simulink model "Continuous_UIO"  (R2021a)
settings: Solver=VariableStepAuto  StartTime=0.0  StopTime=10.0  RelTol=1e-3
values from neighbouring files (symbols this model uses):
  B2 = [4 ... (first row only)    [FunWork5.m]
  D2 = [0 0 ... (first row only)    [FunWork5.m]
  K = Z*S^-1    [FunWork5.m]
  L = X'    [FunWork5.m]
  M = B2*pinv(C*B2)    [FunWork5.m]
  q0 = pi*([x0.x;x0.theta1;x0.theta2;x0.x_dot;x0.theta1_dot;x0.theta2_dot]-x_e)    [FunWork5.m]
undefined symbols (not defined in the file or in its folder): A, B, C, u_e, x0, x_e
libraries: vrlib x2, aerolibanimutils x1, dspvision x1
settings Model: Creator=vicen  LastModifiedBy=vicen

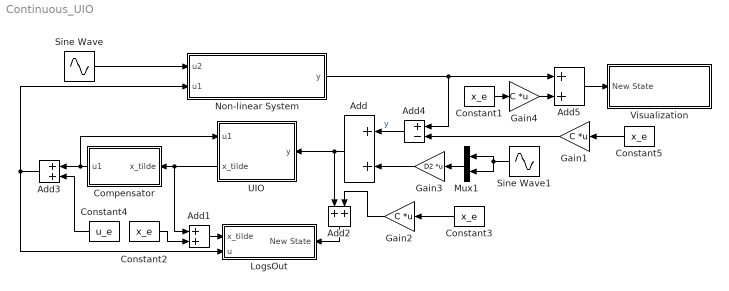
== system Continuous_UIO ==
  Add{,1..3,5} (5 alike) : Sum
  Add4 : Sum  Inputs=+-
  Compensator : Subsystem
  Constant{1..3,5} (4 alike) : Constant  Value=x_e
  Constant4 : Constant  Value=u_e
  Gain1 : Gain  Gain=C  Multiplication=Matrix(K*u)
  Gain2 : Gain  Gain=C  Multiplication=Matrix(K*u)
  Gain3 : Gain  Gain=D2  Multiplication=Matrix(K*u)
  Gain4 : Gain  Gain=C  Multiplication=Matrix(K*u)
  LogsOut : Subsystem
      settings: PortSchema="{\"entries\":[{\"content\":{\"sides\":[{\"content\":{\"connectorIds\":[\"In1\",\"In2\"]},\"type\":\"ConnectorPlacement.EquallySpacedRectSide\",\"uuid\":\"a6e5c360-9678-424a-aca2-159feab9ca2f\"},{\"content\":{\"connectorIds\":[\"In3\"],\"side\":\"RIGHT\"},\"type\":\"ConnectorPlacement.EquallySpacedRectSide\",\"uuid\":\"87be8f2e-6499-443d-a388-19aeb21b3c40\"},{\"content\":{\"connectorIds\":[],\"side\":\"TOP\"},\"type\":\"ConnectorPlacement.EquallySpacedRectSide\",\"uuid\":\"16b12663-65e7-4c0d-a383-2b4d1475174c\"}]},\"type\":\"ConnectorPlacement.EquallySpacedConnector\",\"uuid\":\"7c26d127-e336-47cd-9b3d-f4001f849349\"}],\"packageUris\":[\"http://schema.mathworks.com/mf0/Connector/R2020b\"],\"version\":\"1.0\"}"
  Mux1 : Mux  Inputs=2
  Non-linear System : Subsystem
  Sine Wave : Sin  Amplitude=.001  SampleTime=0
  Sine Wave1 : Sin  Amplitude=.001  SampleTime=0
  UIO : Subsystem
      settings: PortSchema="{\"entries\":[{\"content\":{\"sides\":[{\"content\":{\"connectorIds\":[\"In1\"]},\"type\":\"ConnectorPlacement.EquallySpacedRectSide\",\"uuid\":\"e0fdc8c6-333c-4d3c-a4a6-b3300e16a61f\"},{\"content\":{\"connectorIds\":[\"In2\",\"Out1\"],\"side\":\"RIGHT\"},\"type\":\"ConnectorPlacement.EquallySpacedRectSide\",\"uuid\":\"dbf4194e-4b72-4f2d-9e59-4d14081d6aaf\"},{\"content\":{\"connectorIds\":[],\"side\":\"TOP\"},\"type\":\"ConnectorPlacement.EquallySpacedRectSide\",\"uuid\":\"2ba0a26c-1285-47ee-b6f8-efca2049e722\"}]},\"type\":\"ConnectorPlacement.EquallySpacedConnector\",\"uuid\":\"ed710a6f-1694-499a-b832-87fa0fefc432\"}],\"packageUris\":[\"http://schema.mathworks.com/mf0/Connector/R2020b\"],\"version\":\"1.0\"}"
  Visualization : Subsystem
  wires:
  UIO/1(x_tilde) -> Compensator/1(x_tilde), Add1/1
  Gain3/1 -> Add/2
  Sine Wave1/1 -> Mux1/2, Mux1/1
  Sine Wave/1 -> Non-linear System/1(u2)
  Non-linear System/1(y) -> Add4/1, Add5/1
  Constant2/1 -> Add1/2
  Add1/1 -> LogsOut/1(x_tilde)
  Add/1 -> UIO/1(y), Add2/1
  Constant3/1 -> Gain2/1
  Add2/1 -> LogsOut/3(New State)
  Constant4/1 -> Add3/2
  Compensator/1(u1) -> Add3/1, UIO/2(u1)
  Add3/1 -> Non-linear System/2(u1), LogsOut/2(u)
  Constant5/1 -> Gain1/1
  Add4/1 -> Add/1  "y"
  Gain1/1 -> Add4/2
  Mux1/1 -> Gain3/1
  Gain2/1 -> Add2/2
  Gain4/1 -> Add5/2
  Constant1/1 -> Gain4/1
  Add5/1 -> Visualization/1(New State)

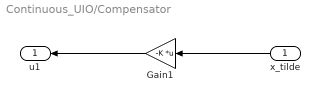
== system Continuous_UIO/Compensator ==
  x_tilde : Inport
  Gain1 : Gain  Gain=-K  Multiplication=Matrix(K*u)
  u1 : Outport
  wires:
  x_tilde/1 -> Gain1/1
  Gain1/1 -> u1/1

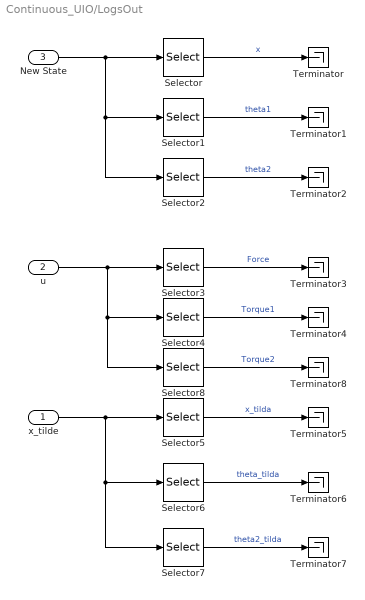
== system Continuous_UIO/LogsOut ==
  x_tilde : Inport
  u : Inport  Port=2
  New State : Inport  Port=3
  Selector : Selector  InputPortWidth=3  IndexOptions=Index vector (dialog)  Indices=1  OutputSizes=1
  Selector1 : Selector  InputPortWidth=3  IndexOptions=Index vector (dialog)  Indices=2  OutputSizes=1
  Selector2 : Selector  InputPortWidth=3  IndexOptions=Index vector (dialog)  Indices=3  OutputSizes=1
  Selector3 : Selector  InputPortWidth=3  IndexOptions=Index vector (dialog)  Indices=1  OutputSizes=1
  Selector4 : Selector  InputPortWidth=3  IndexOptions=Index vector (dialog)  Indices=2  OutputSizes=1
  Selector5 : Selector  InputPortWidth=6  IndexOptions=Index vector (dialog)  Indices=1  OutputSizes=1
  Selector6 : Selector  InputPortWidth=6  IndexOptions=Index vector (dialog)  Indices=2  OutputSizes=1
  Selector7 : Selector  InputPortWidth=6  IndexOptions=Index vector (dialog)  Indices=3  OutputSizes=1
  Selector8 : Selector  InputPortWidth=3  IndexOptions=Index vector (dialog)  Indices=3  OutputSizes=1
  Terminator{,1..8} (9 alike) : Terminator
  wires:
  Selector/1 -> Terminator/1  "x"
  Selector1/1 -> Terminator1/1  "theta1"
  Selector2/1 -> Terminator2/1  "theta2"
  New State/1 -> Selector2/1, Selector1/1, Selector/1
  u/1 -> Selector8/1, Selector4/1, Selector3/1
  Selector4/1 -> Terminator4/1  "Torque1"
  Selector3/1 -> Terminator3/1  "Force"
  x_tilde/1 -> Selector5/1, Selector7/1, Selector6/1
  Selector5/1 -> Terminator5/1  "x_tilda"
  Selector6/1 -> Terminator6/1  "theta_tilda"
  Selector7/1 -> Terminator7/1  "theta2_tilda"
  Selector8/1 -> Terminator8/1  "Torque2"

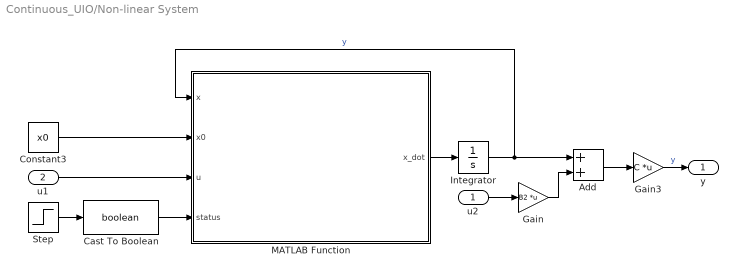
== system Continuous_UIO/Non-linear System ==
  u2 : Inport
  u1 : Inport  Port=2
  Add : Sum
  Cast To Boolean : DataTypeConversion  OutDataTypeStr=boolean
  Constant3 : Constant  Value=x0  VectorParams1D=off  OutDataTypeStr=Bus: State_bus
  Gain : Gain  Gain=B2  Multiplication=Matrix(K*u)
  Gain3 : Gain  Gain=C  Multiplication=Matrix(K*u)
  Integrator : Integrator  InitialCondition=[x0.x;x0.theta1;x0.theta2;x0.x_dot;x0.theta1_dot;x0.theta2_dot]
  MATLAB Function : MATLAB Function  TreatAsAtomicUnit=on
  Step : Step  Time=.001  SampleTime=0
  y : Outport
  wires:
  u1/1 -> MATLAB Function/3(u)
  Step/1 -> Cast To Boolean/1
  Cast To Boolean/1 -> MATLAB Function/4(status)
  Integrator/1 -> Add/1, MATLAB Function/1(x)  "y"
  Constant3/1 -> MATLAB Function/2(x0)
  u2/1 -> Gain/1
  Gain/1 -> Add/2
  MATLAB Function/1(x_dot) -> Integrator/1
  Add/1 -> Gain3/1
  Gain3/1 -> y/1  "y"

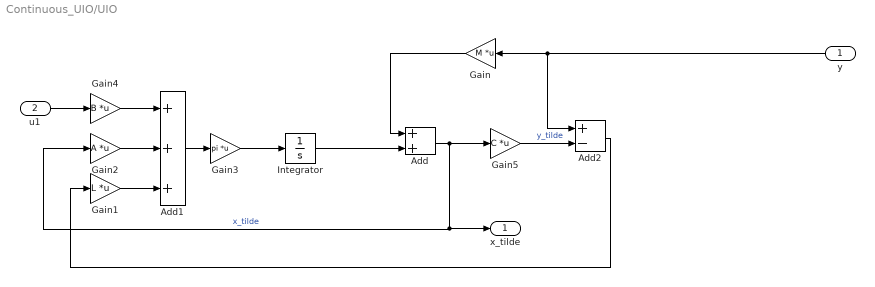
== system Continuous_UIO/UIO ==
  y : Inport
  u1 : Inport  Port=2
  Add : Sum
  Add1 : Sum  Inputs=+++
  Add2 : Sum  Inputs=+-
  Gain : Gain  Gain=M  Multiplication=Matrix(K*u)
  Gain1 : Gain  Gain=L  Multiplication=Matrix(K*u)
  Gain2 : Gain  Gain=A  Multiplication=Matrix(K*u)
  Gain3 : Gain  Gain=pi  Multiplication=Matrix(K*u)
  Gain4 : Gain  Gain=B  Multiplication=Matrix(K*u)
  Gain5 : Gain  Gain=C  Multiplication=Matrix(K*u)
  Integrator : Integrator  InitialCondition=q0
  x_tilde : Outport
  wires:
  Gain/1 -> Add/1
  y/1 -> Gain/1, Add2/1
  u1/1 -> Gain4/1
  Gain4/1 -> Add1/1
  Add1/1 -> Gain3/1
  Integrator/1 -> Add/2
  Add/1 -> Gain2/1, x_tilde/1, Gain5/1  "x_tilde"
  Gain5/1 -> Add2/2  "y_tilde"
  Add2/1 -> Gain1/1
  Gain2/1 -> Add1/2
  Gain1/1 -> Add1/3
  Gain3/1 -> Integrator/1

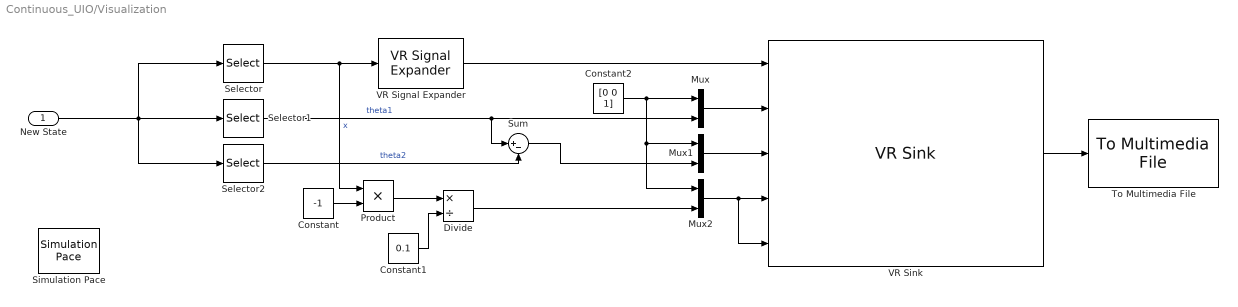
== system Continuous_UIO/Visualization ==
  New State : Inport
  Constant : Constant  Value=-1
  Constant1 : Constant  Value=0.1
  Constant2 : Constant  Value=[0 0 1]
  Divide : Product  Inputs=*/
  Mux : Mux  Inputs=2
  Mux1 : Mux  Inputs=2
  Mux2 : Mux  Inputs=2
  Product : Product
  Selector : Selector  InputPortWidth=3  IndexOptions=Index vector (dialog)  Indices=1  OutputSizes=1
  Selector1 : Selector  InputPortWidth=3  IndexOptions=Index vector (dialog)  Indices=2  OutputSizes=1
  Selector2 : Selector  InputPortWidth=3  IndexOptions=Index vector (dialog)  Indices=3  OutputSizes=1
  Simulation Pace : aerolibanimutils/Simulation Pace  SimulationPace=1  SleepMode=Auto  OutputPaceError=off  SampleTime=1/30
  Sum : Sum  Inputs=|+-
  To Multimedia File : dspvision/To Multimedia File  outputFilename=output2.avi  streamSelection=Video only  videoCompressor=None (uncompressed)  audioCompressor=None (uncompressed)  imagePorts=One multidimensional signal  fileType=AVI  audioDatatype=Determine from input data type  fourcc=RGB  videoQuality=75  mj2000CompFactor=10
  VR Signal Expander : vrlib/VR Signal Expander  outwidth=3  outidx=[1]
  VR Sink : vrlib/VR Sink  InstantiateOnLoad=on  SampleTime=0.1  ViewEnable=on  RemoteChange=off  RemoteView=off  FieldsWritten=Cart.translation.3.1.1.double#Rotation1.rotation.4.1.1.double#Rotation2.rotation.4.1.1.double#Axis_Rotate.rotation.4.1.1.double#Axis_Rotate2.rotation.4.1.1.double  WorldFileName=Cart_Actual.WRL  AutoView=off  VideoDimensions=[1500 2000]  AllowVariableSize=off  FigureProperties="{'Position', 'Name', 'Viewpoint', 'CameraBound', 'CameraDirection', 'CameraPosition', 'CameraUpVector', 'ZoomFactor', 'Antialiasing', 'Headlight', 'Lighting', 'NavPanel', 'Sound', 'StatusBar', 'Stereo3D', 'Stereo3DCameraOffset', 'Stereo3DHIT', 'ToolBar', 'Textures', 'Transparency', 'Triad', 'Wireframe', 'NavZones', 'NavMode', 'NavSpeed', 'CaptureFileFormat', 'CaptureFileName', 'Record2DCompressMethod', 'Record2DCompressQuality', 'Record2D', 'Record2DFileName', 'Record2DFPS'; [1.2660000000000001e+02   9.4799999999999955e+01   8.0000000000000000e+02   6.0020000000000005e+02], '', '_untitled_1', 'on', [0.0000000000000000e+00   0.0000000000000000e+00  -1.0000000000000000e+00], [0.0000000000000000e+00   0.0000000000000000e+00   0.0000000000000000e+00], [0.0000000000000000e+00   1.0000000000000000e+00   0.0000000000000000e+00], [1.0000000000000000e+00], 'on', 'on', 'on', 'none', 'on', 'off', 'off', [1.0000000149011612e-01], [0.0000000000000000e+00], 'off', 'on', 'on', 'none', 'off', 'off', 'fly', 'normal', 'tif', '%f_anim_%n.tif', 'auto', [7.5000000000000000e+01], 'off', '***video***', 'auto'}"
  wires:
  New State/1 -> Selector/1, Selector2/1, Selector1/1
  Selector/1 -> VR Signal Expander/1, Product/1  "x"
  Selector1/1 -> Sum/1, Mux/2  "theta1"
  Product/1 -> Divide/1
  Constant/1 -> Product/2
  Constant1/1 -> Divide/2
  Constant2/1 -> Mux1/1, Mux2/1, Mux/1
  Selector2/1 -> Sum/2  "theta2"
  Divide/1 -> Mux2/2
  Sum/1 -> Mux1/2
  VR Signal Expander/1 -> VR Sink/1
  Mux/1 -> VR Sink/2
  Mux1/1 -> VR Sink/3
  Mux2/1 -> VR Sink/4, VR Sink/5
  VR Sink/1 -> To Multimedia File/1

== matlab function Continuous_UIO/Non-linear System/MATLAB Function ==
  data: x input; x0 input; u input; x_dot output; status input
function x_dot  = Nonlinear_Dynamics(x,x0,u,status)
    if status == false
        x2 = x0.theta1;
        x3 = x0.theta2;
        x4 = x0.x_dot;
        x5 = x0.theta1_dot;
        x6 = x0.theta2_dot;
        u1 = u(1);
        u2 = u(2);
        u3 = u(3);
    else
        x2 = x(2);
        x3 = x(3);
        x4 = x(4);
        x5 = x(5);
        x6 = x(6);
        u1 = u(1);
        u2 = u(2);
        u3 = u(3);
    end
    % Insert Equations
    x_dot = double([
                     x4;
                     x5;
                     x6;
                     -(420*u1 - (2943*sin(2*x2))/2 + 150*x5^2*sin(x2) + (135*x6^2*sin(x3))/2 - 180*u1*cos(2*x2 - 2*x3) + 400*u3*cos(2*x2 - x3) - 840*u2*cos(x2) + 840*u3*cos(x2) - 400*u3*cos(x3) + (135*x6^2*sin(2*x2 - x3))/2 + 360*u2*cos(x2 - 2*x3) - 360*u3*cos(x2 - 2*x3))/(30*(5*cos(2*x2) + 9*cos(2*x2 - 2*x3) - 26));
                     (22800*u3 - 22800*u2 - 26487*sin(x2 - 2*x3) - 91233*sin(x2) + 3600*u2*cos(2*x3) - 3600*u3*cos(2*x3) + 4725*x6^2*sin(x2 - x3) + 750*x5^2*sin(2*x2) - 4000*u3*cos(x2 + x3) + 4200*u1*cos(x2) + 1350*x5^2*sin(2*x2 - 2*x3) - 1800*u1*cos(x2 - 2*x3) + 13600*u3*cos(x2 - x3) + 675*x6^2*sin(x2 + x3))/(150*(5*cos(2*x2) + 9*cos(2*x2 - 2*x3) - 26));
                     -(2700*sin(x2 - x3)*x5^2 + 1215*sin(2*x2 - 2*x3)*x6^2 + 13600*u3 - 26487*sin(2*x2 - x3) + 26487*sin(x3) - 4000*u3*cos(2*x2) + 1800*u1*cos(2*x2 - x3) + 3600*u2*cos(x2 + x3) - 3600*u3*cos(x2 + x3) - 1800*u1*cos(x3) - 12240*u2*cos(x2 - x3) + 12240*u3*cos(x2 - x3))/(135*(5*cos(2*x2) + 9*cos(2*x2 - 2*x3) - 26))
                ]);
            
end
